simulink model "iLQCsimulation"  (R2025a)
settings: Solver=FixedStepAuto  StartTime=0.0  StopTime=20  FixedStep=0.01  RelTol=1e-3
StopFcn:
  | fprintf("Done\n");
values from neighbouring files (symbols this model uses):
  cmd = permute(cat(3, theta_ff', permute(theta_fb, [3, 1, 2])), [2, 3, 1])    [run_iLQR_simulation.m]
undefined symbols (not defined in the file or in its folder): ics, it, params, sim_, WpNav_hdg, WpNav_pos, WpNav_spd
libraries: matrix_library x1, sharedutil x1, sharedtransform x1, dspinverses x1
settings Model: Creator=Cindio  LastModifiedBy=cfeng
settings DataIOCC: SignalLogging=off  DSMLogging=off  ReturnWorkspaceOutputs=off
settings ModelReferenceCC: EnableRefExpFcnMdlSchedulingChecks=on
settings RTWCC: GPUComputeCapability=3.5  DLArmComputeVersion=19.05

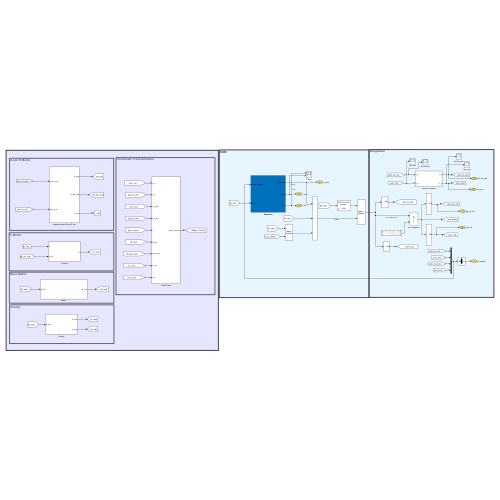
[thumbnail: Simulink's stored preview of the top-level diagram]
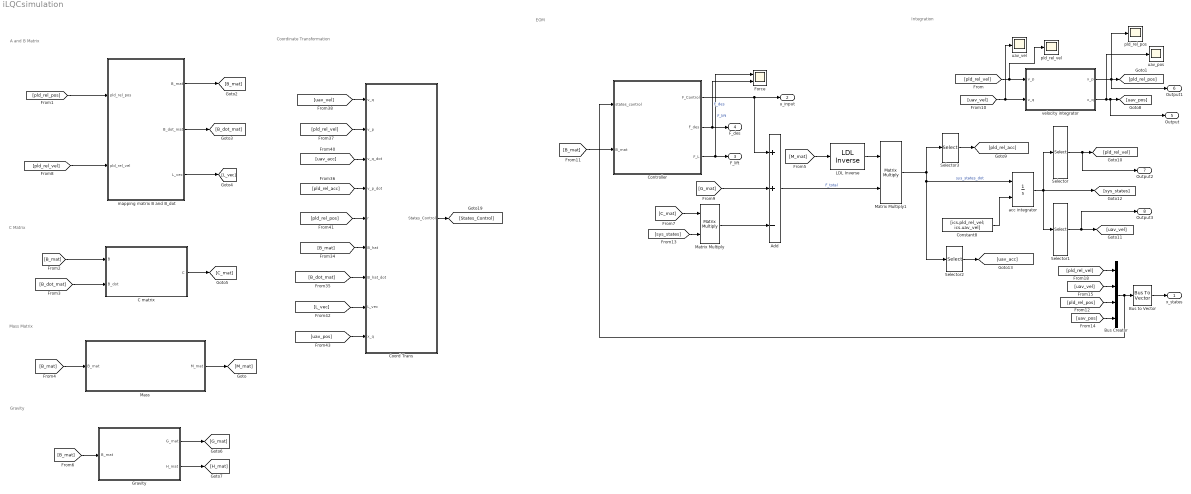
== system iLQCsimulation ==
  note: Integration
  note: EOM
  note: Gravity
  note: Mass Matrix
  note: C Matrix
  note: A and B Matrix
  note: Coordinate Transformation
  Add : Sum  Inputs=++-
  Bus Creator : BusCreator  Inputs=4
  Bus to Vector : BusToVector
  C matrix : Subsystem
  Constant8 : Constant  Value=[ics.pld_rel_vel; ics.uav_vel]  VectorParams1D=off
  Controller : Subsystem
  Coord Trans : Subsystem
  Force : Scope  NumInputPorts=2
      settings: ActiveDisplayYMinimum=-50.13137  ActiveDisplayYMaximum=10.24437
  Gravity : Subsystem
  LDL Inverse : dspinverses/LDL Inverse  errmode=Error
  Mass : Subsystem
  Matrix Multiply : Product  Multiplication=Matrix(*)
  Matrix Multiply1 : Product  Multiplication=Matrix(*)
  Selector : Selector  InputPortWidth=5  IndexOptions=Index vector (dialog)  Indices=[1 2]  OutputSizes=1
  Selector1 : Selector  InputPortWidth=5  IndexOptions=Index vector (dialog)  Indices=[3 4 5]  OutputSizes=1
  Selector2 : Selector  InputPortWidth=5  IndexOptions=Index vector (dialog)  Indices=[3 4 5]  OutputSizes=1
  Selector3 : Selector  InputPortWidth=5  IndexOptions=Index vector (dialog)  Indices=[1 2]  OutputSizes=1
  acc integrator : Integrator  InitialConditionSource=external
  mapping matrix B and B_dot : Subsystem
  pld_rel_pos : Scope
      settings: Title=Payload relative position  ActiveDisplayYMinimum=-0.0462  ActiveDisplayYMaximum=0.05217  YLabel=position (m)
  pld_rel_vel : Scope
      settings: Title=UAV Position  ActiveDisplayYMinimum=-0.10534  ActiveDisplayYMaximum=0.12291  YLabel=position (m)
  uav_pos : Scope
      settings: Title=UAV Position  ActiveDisplayYMinimum=-3.62298  ActiveDisplayYMaximum=2.12156  YLabel=position (m)  DataLoggingVariableName=ScopeData2
  uav_vel : Scope
      settings: Title=UAV Velocity  ActiveDisplayYMinimum=-0.42187  ActiveDisplayYMaximum=0.54304  YLabel=speed (m/s)  DataLoggingVariableName=ScopeData2
  velocity integrator : Subsystem
  x_states : Outport  SignalName=all_states
  u_input : Outport  Port=2  SignalName=u_input
  F_lift : Outport  Port=3  SignalName=F_lift
  F_des : Outport  Port=4  SignalName=F_des
  Output : Outport  Port=5  SignalName=uav_pos
  Output1 : Outport  Port=6  SignalName=pld_rel_pos
  Output2 : Outport  Port=7  SignalName=pld_rel_vel
  Output3 : Outport  Port=8  SignalName=uav_vel
  wires:
  [pld_rel_vel] -> pld_rel_vel/1, velocity integrator/1(v_p)
  velocity integrator/1(x_p) -> Output1/1, pld_rel_pos/1, [pld_rel_pos]
  mapping matrix B and B_dot/1(B_mat) -> [B_mat]
  mapping matrix B and B_dot/2(B_dot_mat) -> [B_dot_mat]
  mapping matrix B and B_dot/3(L_vec) -> [L_vec]
  [B_dot_mat] -> C matrix/2(B_dot)
  C matrix/1(C) -> [C_mat]
  [B_mat] -> Mass/1(B_mat)
  Mass/1(M_mat) -> [M_mat]
  [M_mat] -> LDL Inverse/1
  [B_mat] -> Gravity/1(B_mat)
  Gravity/2(H_mat) -> [H_mat]
  Matrix Multiply/1 -> Add/3
  [G_mat] -> Add/2
  Gravity/1(G_mat) -> [G_mat]
  [pld_rel_pos] -> mapping matrix B and B_dot/1(pld_rel_pos)
  [C_mat] -> Matrix Multiply/1
  [pld_rel_vel] -> mapping matrix B and B_dot/2(pld_rel_vel)
  [uav_vel] -> uav_vel/1, velocity integrator/2(v_q)
  [sys_states] -> Matrix Multiply/2
  LDL Inverse/1 -> Matrix Multiply1/1
  Add/1 -> Matrix Multiply1/2  "F_total"
  Matrix Multiply1/1 -> Selector3/1, Selector2/1, acc integrator/1  "sys_states_dot"
  Constant8/1 -> acc integrator/2
  acc integrator/1 -> Selector1/1, [sys_states], Selector/1
  Selector/1 -> Output2/1, [pld_rel_vel]
  Selector1/1 -> Output3/1, [uav_vel]
  [B_dot_mat] -> Coord Trans/7(B_hat_dot)
  [uav_vel] -> Coord Trans/1(v_q)
  [pld_rel_vel] -> Coord Trans/2(v_p)
  Coord Trans/1(States_Control) -> [States_Control]
  [B_mat] -> Coord Trans/6(B_hat)
  [pld_rel_pos] -> Coord Trans/5(r)
  [uav_pos] -> Coord Trans/9(x_q)
  [L_vec] -> Coord Trans/8(L_vec)
  [uav_acc] -> Coord Trans/3(v_q_dot)
  [pld_rel_acc] -> Coord Trans/4(v_p_dot)
  Selector3/1 -> [pld_rel_acc]
  Selector2/1 -> [uav_acc]
  Bus Creator/1 -> Bus to Vector/1, Controller/1(states_control)
  Controller/1(F_Control) -> Add/1, u_input/1
  velocity integrator/2(x_q) -> uav_pos/1, Output/1, [uav_pos]
  [pld_rel_pos] -> Bus Creator/3
  [uav_pos] -> Bus Creator/4
  [uav_vel] -> Bus Creator/2
  [pld_rel_vel] -> Bus Creator/1
  Bus to Vector/1 -> x_states/1
  [B_mat] -> Controller/2(B_mat)
  Controller/3(F_L) -> Force/1, F_lift/1  "F_lift"
  Controller/2(F_des) -> Force/2, F_des/1  "F_des"
  [B_mat] -> C matrix/1(B)

== system iLQCsimulation/C matrix ==
  B : Inport
  B_dot : Inport  Port=2
  Constant : Constant  Value=[zeros(2,3);zeros(3)]  VectorParams1D=off
  Matrix Concatenate : Concatenate  Mode=Multidimensional array  ConcatenateDimension=2
  Matrix Concatenate1 : Concatenate  Mode=Multidimensional array
  Matrix Multiply : Product  Multiplication=Matrix(*)
  Multiply : Gain  Gain=params.pld_mass
  Transpose : Math  Operator=transpose
  C : Outport
  wires:
  Constant/1 -> Matrix Concatenate/2
  Matrix Concatenate/1 -> C/1
  Matrix Multiply/1 -> Matrix Concatenate1/1
  B/1 -> Transpose/1
  Transpose/1 -> Matrix Multiply/1
  B_dot/1 -> Matrix Concatenate1/2, Matrix Multiply/2
  Multiply/1 -> Matrix Concatenate/1
  Matrix Concatenate1/1 -> Multiply/1

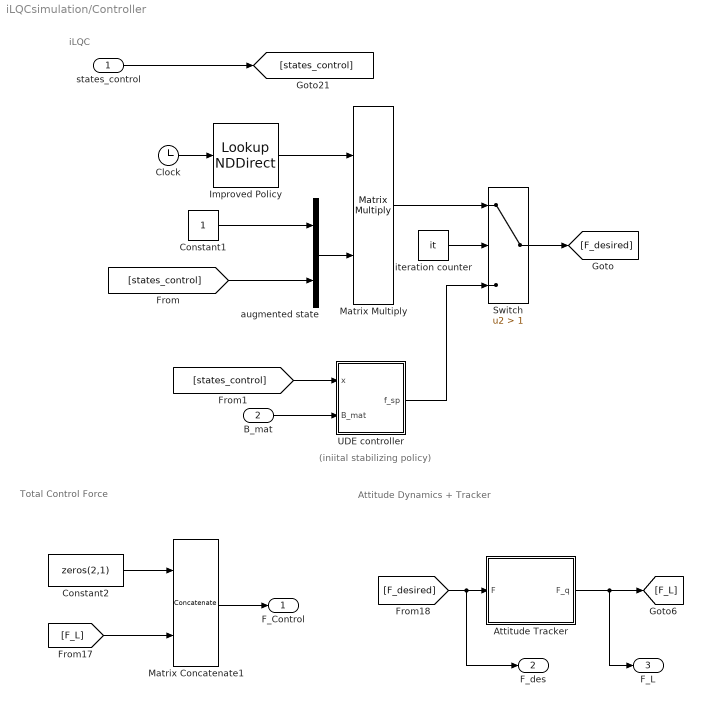
== system iLQCsimulation/Controller ==
  note: (iniital stabilizing policy)
  note: iLQC
  note: Total Control Force
  note: Attitude Dynamics + Tracker
  states_control : Inport
  B_mat : Inport  Port=2
  Attitude Tracker : Subsystem
  Clock : Clock
  Constant1 : Constant
  Constant2 : Constant  Value=zeros(2,1)
  Improved Policy : LookupNDDirect  NumberOfTableDimensions=3  InputsSelectThisObjectFromTable=2-D Matrix  Table=cmd  DiagnosticForOutOfRangeInput=Error
  Matrix Concatenate1 : Concatenate  Mode=Multidimensional array
  Matrix Multiply : Product  Multiplication=Matrix(*)
  Switch : Switch  Criteria=u2 > Threshold  Threshold=1  SaturateOnIntegerOverflow=off  InputSameDT=off
  "UDE controller " : Subsystem
  augmented state : Concatenate
  iteration counter : Constant  Value=it
  F_Control : Outport  VectorParamsAs1DForOutWhenUnconnected=off
  F_des : Outport  Port=2  VectorParamsAs1DForOutWhenUnconnected=off
  F_L : Outport  Port=3  VectorParamsAs1DForOutWhenUnconnected=off
  wires:
  Constant2/1 -> Matrix Concatenate1/1
  Matrix Concatenate1/1 -> F_Control/1
  [F_L] -> Matrix Concatenate1/2
  Attitude Tracker/1(F_q) -> F_L/1, [F_L]
  [F_desired] -> F_des/1, Attitude Tracker/1(F)
  Improved Policy/1 -> Matrix Multiply/1
  Clock/1 -> Improved Policy/1
  Matrix Multiply/1 -> Switch/1
  Constant1/1 -> augmented state/1
  iteration counter/1 -> Switch/2
  Switch/1 -> [F_desired]
  [states_control] -> "UDE controller "/1(x)
  B_mat/1 -> "UDE controller "/2(B_mat)
  "UDE controller "/1(f_sp) -> Switch/3
  states_control/1 -> [states_control]
  [states_control] -> augmented state/2
  augmented state/1 -> Matrix Multiply/2

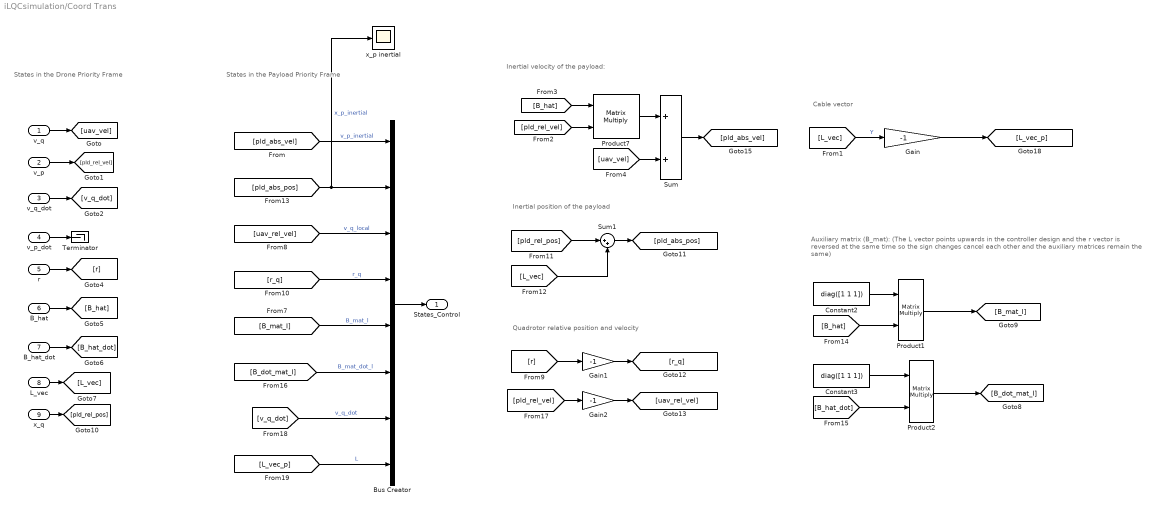
== system iLQCsimulation/Coord Trans ==
  note: Quadrotor relative position and velocity
  note: Auxiliary matrix (B_mat):
      | (The L vector points upwards in the controller design and the r vector is reversed at the same time so the sign changes cancel each other and the auxiliary matrices remain the same)
  note: Inertial position of the payload
  note: Cable vector
  note: Inertial velocity of the payload:
  note: States in the Drone Priority Frame
  note: States in the Payload Priority Frame
  v_q : Inport
  v_p : Inport  Port=2
  v_q_dot : Inport  Port=3
  v_p_dot : Inport  Port=4
  r : Inport  Port=5
  B_hat : Inport  Port=6
  B_hat_dot : Inport  Port=7
  L_vec : Inport  Port=8
  x_q : Inport  Port=9
  Bus Creator : BusCreator  Inputs=8
  Constant2 : Constant  Value=diag([1 1 1])
  Constant3 : Constant  Value=diag([1 1 1])
  Gain : Gain  Gain=-1
  Gain1 : Gain  Gain=-1
  Gain2 : Gain  Gain=-1
  Product1 : Product  Multiplication=Matrix(*)
  Product2 : Product  Multiplication=Matrix(*)
  Product7 : Product  Multiplication=Matrix(*)
  Sum : Sum
  Sum1 : Sum  Inputs=|++
  Terminator : Terminator
  x_p inertial : Scope
      settings: ActiveDisplayYMinimum=-3.375  ActiveDisplayYMaximum=0.375
  States_Control : Outport  VectorParamsAs1DForOutWhenUnconnected=off
  wires:
  Bus Creator/1 -> States_Control/1
  Product7/1 -> Sum/1
  Sum/1 -> [pld_abs_vel]
  [uav_vel] -> Sum/2
  [L_vec] -> Gain/1  "Y"
  Gain/1 -> [L_vec_p]
  v_q/1 -> [uav_vel]
  v_p/1 -> [pld_rel_vel]
  v_q_dot/1 -> [v_q_dot]
  v_p_dot/1 -> Terminator/1
  r/1 -> [r]
  B_hat/1 -> [B_hat]
  B_hat_dot/1 -> [B_hat_dot]
  L_vec/1 -> [L_vec]
  x_q/1 -> [pld_rel_pos]
  [pld_rel_pos] -> Sum1/1
  [L_vec] -> Sum1/2
  Sum1/1 -> [pld_abs_pos]
  [r] -> Gain1/1
  Gain1/1 -> [r_q]
  [pld_abs_vel] -> Bus Creator/1  "v_p_inertial"
  [pld_abs_pos] -> x_p inertial/1, Bus Creator/2  "x_p_inertial"
  [uav_rel_vel] -> Bus Creator/3  "v_q_local"
  [r_q] -> Bus Creator/4  "r_q"
  [B_mat_I] -> Bus Creator/5  "B_mat_l"
  [B_dot_mat_I] -> Bus Creator/6  "B_mat_dot_l"
  [B_hat] -> Product1/2
  Product1/1 -> [B_mat_I]
  [B_hat_dot] -> Product2/2
  Product2/1 -> [B_dot_mat_I]
  [pld_rel_vel] -> Gain2/1
  Gain2/1 -> [uav_rel_vel]
  [v_q_dot] -> Bus Creator/7  "v_q_dot"
  [L_vec_p] -> Bus Creator/8  "L"
  [pld_rel_vel] -> Product7/2
  [B_hat] -> Product7/1
  Constant2/1 -> Product1/1
  Constant3/1 -> Product2/1

== system iLQCsimulation/Gravity ==
  B_mat : Inport
  Constant : Constant  Value=zeros(2,3)  VectorParams1D=off
  Constant1 : Constant  Value=[eye(3),eye(3)]  VectorParams1D=off
  Constant2 : Constant  Value=params.derived.uav_weight
  Constant3 : Constant  Value=params.derived.pld_weight
  Matrix Concatenate : Concatenate  Mode=Multidimensional array  ConcatenateDimension=2
  Matrix Concatenate1 : Concatenate  Mode=Multidimensional array
  Matrix Concatenate2 : Concatenate
  Matrix Multiply : Product  Multiplication=Matrix(*)
  Transpose : Math  Operator=transpose
  G_mat : Outport
  H_mat : Outport  Port=2
  wires:
  Constant/1 -> Matrix Concatenate/2
  B_mat/1 -> Transpose/1
  Matrix Concatenate/1 -> Matrix Concatenate1/1
  Constant1/1 -> Matrix Concatenate1/2
  Matrix Concatenate1/1 -> [H], H_mat/1
  [H] -> Matrix Multiply/1
  Matrix Multiply/1 -> G_mat/1
  Matrix Concatenate2/1 -> Matrix Multiply/2
  Constant3/1 -> Matrix Concatenate2/1
  Transpose/1 -> Matrix Concatenate/1
  Constant2/1 -> Matrix Concatenate2/2

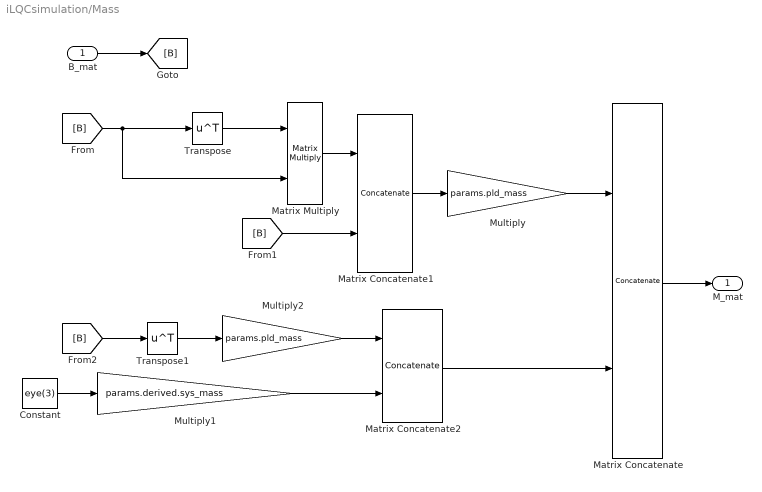
== system iLQCsimulation/Mass ==
  B_mat : Inport
  Constant : Constant  Value=eye(3)
  Matrix Concatenate : Concatenate  Mode=Multidimensional array  ConcatenateDimension=2
  Matrix Concatenate1 : Concatenate  Mode=Multidimensional array
  Matrix Concatenate2 : Concatenate  Mode=Multidimensional array
  Matrix Multiply : Product  Multiplication=Matrix(*)
  Multiply : Gain  Gain=params.pld_mass
  Multiply1 : Gain  Gain=params.derived.sys_mass
  Multiply2 : Gain  Gain=params.pld_mass
  Transpose : Math  Operator=transpose
  Transpose1 : Math  Operator=transpose
  M_mat : Outport
  wires:
  Matrix Concatenate/1 -> M_mat/1
  Matrix Concatenate1/1 -> Multiply/1
  Multiply/1 -> Matrix Concatenate/1
  B_mat/1 -> [B]
  [B] -> Matrix Multiply/2, Transpose/1
  Transpose/1 -> Matrix Multiply/1
  Matrix Multiply/1 -> Matrix Concatenate1/1
  [B] -> Matrix Concatenate1/2
  Constant/1 -> Multiply1/1
  Multiply1/1 -> Matrix Concatenate2/2
  Matrix Concatenate2/1 -> Matrix Concatenate/2
  [B] -> Transpose1/1
  Transpose1/1 -> Multiply2/1
  Multiply2/1 -> Matrix Concatenate2/1

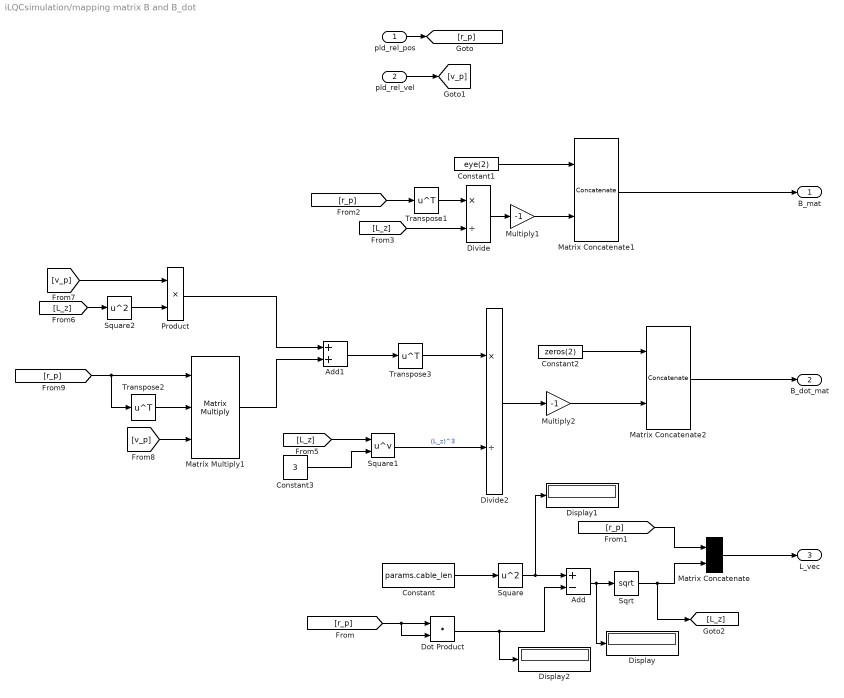
== system iLQCsimulation/mapping matrix B and B_dot ==
  pld_rel_pos : Inport
  pld_rel_vel : Inport  Port=2
  Add : Sum  Inputs=+-
  Add1 : Sum
  Constant : Constant  Value=params.cable_len
  Constant1 : Constant  Value=eye(2)
  Constant2 : Constant  Value=zeros(2)
  Constant3 : Constant  Value=3
  Display : Display
  Display1 : Display
  Display2 : Display
  Divide : Product  Inputs=*/
  Divide2 : Product  Inputs=*/
  Dot Product : DotProduct  OutDataTypeStr=Inherit: Inherit via internal rule
  Matrix Concatenate : Concatenate
  Matrix Concatenate1 : Concatenate  Mode=Multidimensional array
  Matrix Concatenate2 : Concatenate  Mode=Multidimensional array
  Matrix Multiply1 : Product  Inputs=3  Multiplication=Matrix(*)
  Multiply1 : Gain  Gain=-1
  Multiply2 : Gain  Gain=-1
  Product : Product
  Sqrt : Sqrt
  Square : Math  Operator=square
  Square1 : Math  Operator=pow
  Square2 : Math  Operator=square
  Transpose1 : Math  Operator=transpose
  Transpose2 : Math  Operator=transpose
  Transpose3 : Math  Operator=transpose
  B_mat : Outport
  B_dot_mat : Outport  Port=2
  L_vec : Outport  Port=3
  wires:
  Constant/1 -> Square/1
  Square/1 -> Display1/1, Add/1
  pld_rel_pos/1 -> [r_p]
  Add/1 -> Display/1, Sqrt/1
  Sqrt/1 -> [L_z], Matrix Concatenate/2
  [r_p] -> Matrix Concatenate/1
  pld_rel_vel/1 -> [v_p]
  Matrix Concatenate/1 -> L_vec/1
  [r_p] -> Transpose1/1
  Transpose1/1 -> Divide/1
  Constant1/1 -> Matrix Concatenate1/1
  Divide/1 -> Multiply1/1
  [L_z] -> Divide/2
  Multiply1/1 -> Matrix Concatenate1/2
  Matrix Concatenate1/1 -> B_mat/1
  Matrix Concatenate2/1 -> B_dot_mat/1
  Constant2/1 -> Matrix Concatenate2/1
  [L_z] -> Square1/1
  Square1/1 -> Divide2/2  "(L_z)^3"
  [L_z] -> Square2/1
  [v_p] -> Product/1
  Transpose2/1 -> Matrix Multiply1/2
  Matrix Multiply1/1 -> Add1/2
  [r_p] -> Transpose2/1, Matrix Multiply1/1
  [v_p] -> Matrix Multiply1/3
  Constant3/1 -> Square1/2
  Divide2/1 -> Multiply2/1
  Add1/1 -> Transpose3/1
  Product/1 -> Add1/1
  Square2/1 -> Product/2
  [r_p] -> Dot Product/2, Dot Product/1
  Dot Product/1 -> Display2/1, Add/2
  Transpose3/1 -> Divide2/1
  Multiply2/1 -> Matrix Concatenate2/2

== system iLQCsimulation/velocity integrator ==
  v_p : Inport
  v_q : Inport  Port=2
  Constant : Constant  Value=ics.pld_rel_pos
  Constant1 : Constant  Value=ics.uav_pos
  Integrator : Integrator  InitialConditionSource=external
  Integrator1 : Integrator  InitialConditionSource=external
  x_p : Outport
  x_q : Outport  Port=2
  wires:
  Integrator/1 -> x_p/1
  Constant/1 -> Integrator/2
  v_p/1 -> Integrator/1
  Constant1/1 -> Integrator1/2
  v_q/1 -> Integrator1/1
  Integrator1/1 -> x_q/1

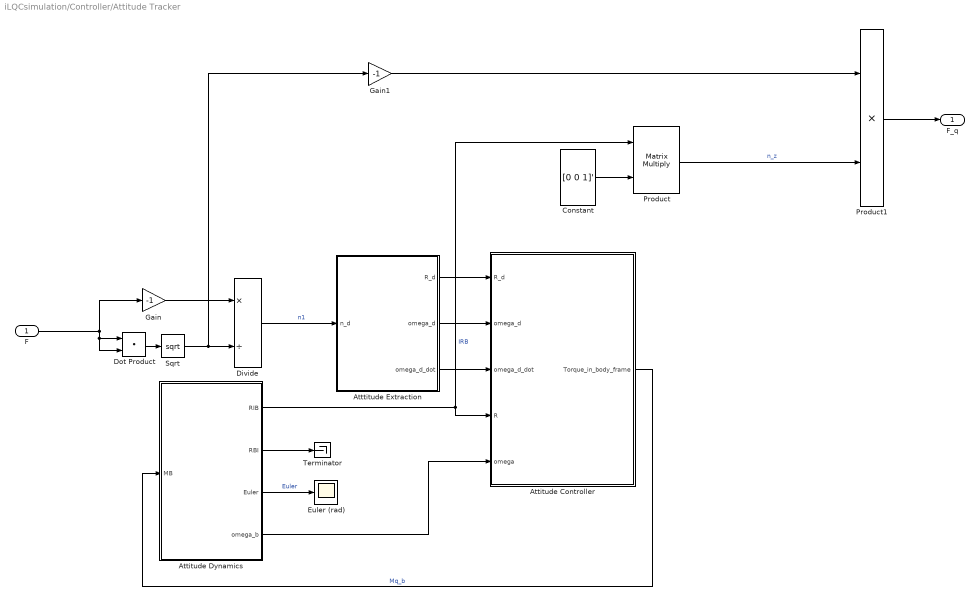
== system iLQCsimulation/Controller/Attitude Tracker ==
  F : Inport
  Attitude Controller : Subsystem
  Attitude Dynamics : Subsystem
  Atttitude Extraction : Subsystem
  Constant : Constant  Value=[0 0 1]'  VectorParams1D=off
  Divide : Product  Inputs=*/
  Dot Product : DotProduct  OutDataTypeStr=Inherit: Inherit via internal rule
  Euler (rad) : Scope
      settings: ActiveDisplayYMinimum=-0.01904  ActiveDisplayYMaximum=0.02201  DataLoggingVariableName=ScopeData2
  Gain : Gain  Gain=-1
  Gain1 : Gain  Gain=-1
  Product : Product  Multiplication=Matrix(*)
  Product1 : Product
  Sqrt : Sqrt
  Terminator : Terminator
  F_q : Outport  VectorParamsAs1DForOutWhenUnconnected=off
  wires:
  Constant/1 -> Product/2
  Product/1 -> Product1/2  "n_z"
  Product1/1 -> F_q/1
  Dot Product/1 -> Sqrt/1
  Atttitude Extraction/1(R_d) -> Attitude Controller/1(R_d)
  Atttitude Extraction/2(omega_d) -> Attitude Controller/2(omega_d)
  Atttitude Extraction/3(omega_d_dot) -> Attitude Controller/3(omega_d_dot)
  Divide/1 -> Atttitude Extraction/1(n_d)  "n1"
  Attitude Dynamics/4(omega_b) -> Attitude Controller/5(omega)
  Attitude Dynamics/3(Euler) -> Euler (rad)/1  "Euler"
  Attitude Dynamics/2(RBI) -> Terminator/1
  Attitude Dynamics/1(RIB) -> Attitude Controller/4(R), Product/1  "IRB"
  Attitude Controller/1(Torque_in_body_frame) -> Attitude Dynamics/1(MB)  "Mq_b"
  F/1 -> Gain/1, Dot Product/2, Dot Product/1
  Sqrt/1 -> Gain1/1, Divide/2
  Gain/1 -> Divide/1
  Gain1/1 -> Product1/1

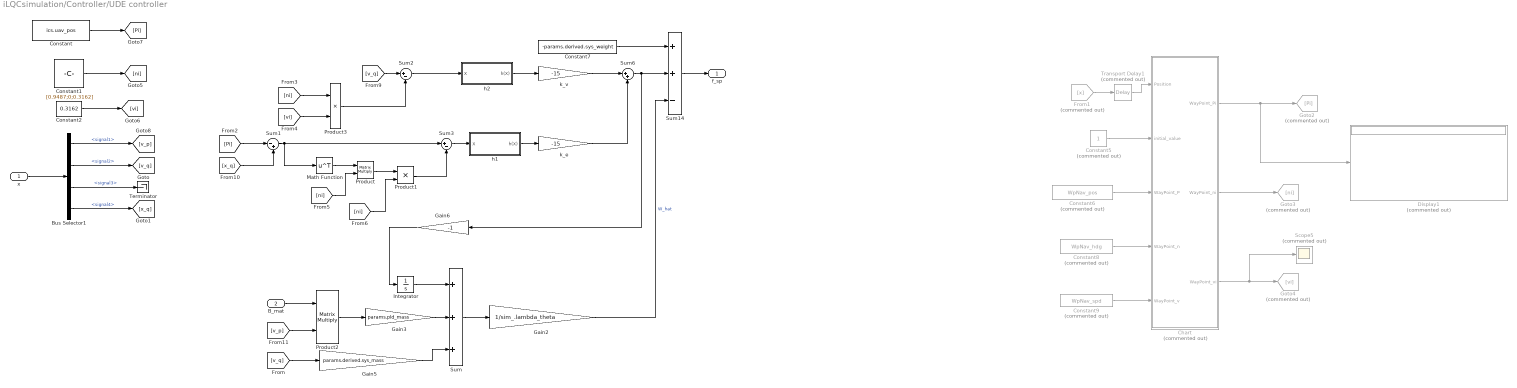
== system iLQCsimulation/Controller/UDE controller  ==
  x : Inport
  B_mat : Inport  Port=2
  Bus Selector1 : BusSelector  OutputSignals=signal1,signal2,signal3,signal4
  Chart : Stateflow chart  Commented=on  TreatAsAtomicUnit=on
  Constant : Constant  Value=ics.uav_pos  VectorParams1D=off
  Constant1 : Constant  Value=[0.9487;0;0.3162]  VectorParams1D=off
  Constant2 : Constant  Value=0.3162
  Constant5 : Constant  Commented=on
  Constant6 : Constant  Commented=on  Value=WpNav_pos
  Constant7 : Constant  Value=-params.derived.sys_weight  VectorParams1D=off
  Constant8 : Constant  Commented=on  Value=WpNav_hdg
  Constant9 : Constant  Commented=on  Value=WpNav_spd
  Display1 : Display  Commented=on
  From1 : From  Commented=on  GotoTag=x
  Gain2 : Gain  Gain=1/sim_.lambda_theta
  Gain3 : Gain  Gain=params.pld_mass
  Gain5 : Gain  Gain=params.derived.sys_mass
  Gain6 : Gain  Gain=-1
  Goto2 : Goto  Commented=on  GotoTag=Pi
  Goto3 : Goto  Commented=on  GotoTag=ni
  Goto4 : Goto  Commented=on  GotoTag=vi
  Integrator : Integrator
  Math Function : Math  Operator=transpose  SignedPower=on
  Product : Product  Multiplication=Matrix(*)
  Product1 : Product
  Product2 : Product  Multiplication=Matrix(*)
  Product3 : Product
  Scope5 : Scope  Commented=on
      settings: ActiveDisplayYMinimum=-1.25  ActiveDisplayYMaximum=11.25  DataLoggingVariableName=ScopeData3
  Sum : Sum  Inputs=+++
  Sum1 : Sum  Inputs=|-+
  Sum14 : Sum  Inputs=++-
  Sum2 : Sum  Inputs=|+-
  Sum3 : Sum  Inputs=|+-
  Sum6 : Sum  Inputs=|++
  Terminator : Terminator
  Transport Delay1 : TransportDelay  Commented=on  DelayTime=0.3
  h1 : Subsystem
  h2 : Subsystem
  k_e : Gain  Gain=-15
  k_v : Gain  Gain=-15
  f_sp : Outport
  wires:
  Sum14/1 -> f_sp/1
  [ni] -> Product3/1
  [Pi] -> Sum1/1
  Product3/1 -> Sum2/2
  h1/1(h(X)) -> k_e/1
  k_e/1 -> Sum6/2
  Sum1/1 -> Math Function/1, Sum3/1
  Math Function/1 -> Product/1
  [ni] -> Product/2
  Product/1 -> Product1/1
  [ni] -> Product1/2
  Product1/1 -> Sum3/2
  k_v/1 -> Sum6/1
  h2/1(h(X)) -> k_v/1
  Sum2/1 -> h2/1(X)
  Sum6/1 -> Gain6/1, Sum14/2
  Constant7/1 -> Sum14/1
  Sum/1 -> Gain2/1
  Bus Selector1/1 -> [v_p]  "<signal1>"
  Product2/1 -> Gain3/1
  [v_q] -> Gain5/1
  Gain3/1 -> Sum/2
  Gain5/1 -> Sum/3
  Integrator/1 -> Sum/1
  Gain6/1 -> Integrator/1
  Gain2/1 -> Sum14/3  "W_hat"
  Constant5/1 -> Chart/2(initial_value)
  From1/1 -> Transport Delay1/1
  Constant6/1 -> Chart/3(WayPoint_P)
  Constant8/1 -> Chart/4(WayPoint_n)
  Constant9/1 -> Chart/5(WayPoint_v)
  [vi] -> Product3/2
  Transport Delay1/1 -> Chart/1(Position)
  Sum3/1 -> h1/1(X)
  Chart/2(WayPoint_ni) -> Goto3/1
  Chart/3(WayPoint_vi) -> Scope5/1, Goto4/1
  Chart/1(WayPoint_Pi) -> Display1/1, Goto2/1
  Bus Selector1/3 -> Terminator/1  "<signal3>"
  x/1 -> Bus Selector1/1
  Constant/1 -> [Pi]
  Constant1/1 -> [ni]
  Constant2/1 -> [vi]
  B_mat/1 -> Product2/1
  Bus Selector1/2 -> [v_q]  "<signal2>"
  [v_q] -> Sum2/1
  Bus Selector1/4 -> [x_q]  "<signal4>"
  [x_q] -> Sum1/2
  [v_p] -> Product2/2

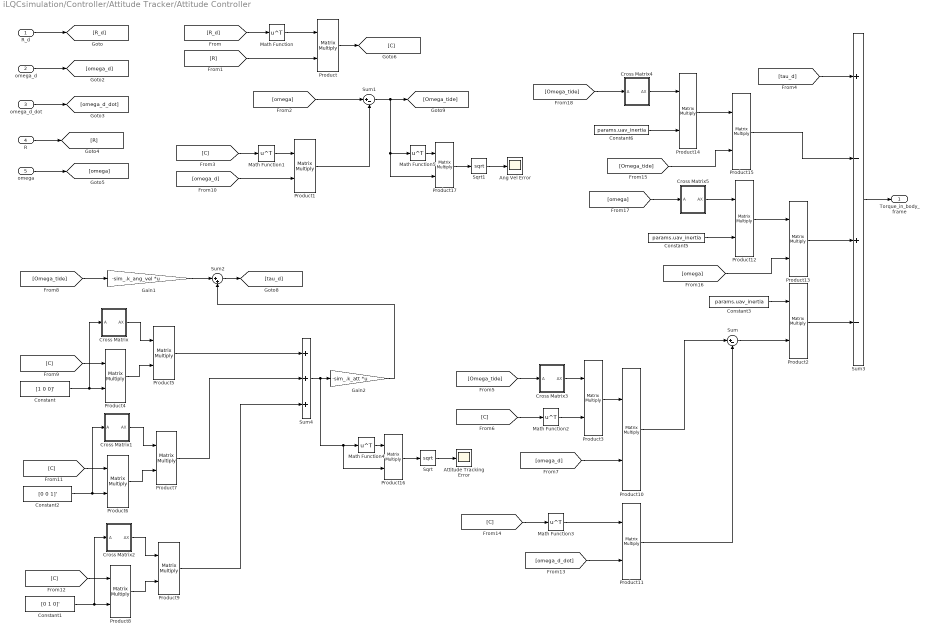
== system iLQCsimulation/Controller/Attitude Tracker/Attitude Controller ==
  R_d : Inport
  omega_d : Inport  Port=2
  omega_d_dot : Inport  Port=3
  R : Inport  Port=4
  omega : Inport  Port=5
  Ang Vel Error : Scope
      settings: ActiveDisplayYMinimum=-1.77018  ActiveDisplayYMaximum=15.93169  DataLoggingVariableName=ScopeData9
  Attitude Tracking Error : Scope
      settings: ActiveDisplayYMinimum=-0.14827  ActiveDisplayYMaximum=1.33442  DataLoggingVariableName=ScopeData10
  Constant : Constant  Value=[1 0 0]'
  Constant1 : Constant  Value=[0 1 0]'
  Constant2 : Constant  Value=[0 0 1]'
  Constant3 : Constant  Value=params.uav_inertia  VectorParams1D=off
  Constant5 : Constant  Value=params.uav_inertia  VectorParams1D=off
  Constant6 : Constant  Value=params.uav_inertia  VectorParams1D=off
  Cross Matrix : Subsystem
  Cross Matrix1 : Subsystem
  Cross Matrix2 : Subsystem
  Cross Matrix3 : Subsystem
  Cross Matrix4 : Subsystem
  Cross Matrix5 : Subsystem
  Gain1 : Gain  Gain=-sim_.k_ang_vel  Multiplication=Matrix(K*u)
  Gain2 : Gain  Gain=-sim_.k_att  Multiplication=Matrix(K*u)
  Math Function{,1..5} (6 alike) : Math  Operator=transpose  SignedPower=on
  Product{,1..17} (18 alike) : Product  Multiplication=Matrix(*)
  Sqrt : Sqrt
  Sqrt1 : Sqrt
  Sum : Sum  Inputs=|+-
  Sum1 : Sum  Inputs=|+-
  Sum2 : Sum  Inputs=|++
  Sum3 : Sum  Inputs=+-+-
  Sum4 : Sum  Inputs=+++
  Torque_in_body_frame : Outport  VectorParamsAs1DForOutWhenUnconnected=off
  wires:
  R_d/1 -> [R_d]
  omega_d/1 -> [omega_d]
  omega_d_dot/1 -> [omega_d_dot]
  [R_d] -> Math Function/1
  Math Function/1 -> Product/1
  R/1 -> [R]
  omega/1 -> [omega]
  [R] -> Product/2
  Product/1 -> [C]
  [C] -> Math Function1/1
  Math Function1/1 -> Product1/1
  [omega] -> Sum1/1
  Product1/1 -> Sum1/2
  [omega_d] -> Product1/2
  Sum2/1 -> [tau_d]
  Gain1/1 -> Sum2/1
  [Omega_tide] -> Gain1/1
  [tau_d] -> Sum3/1
  [C] -> Product4/1
  Constant/1 -> Cross Matrix/1(A), Product4/2
  Cross Matrix/1(AX) -> Product5/1
  Product4/1 -> Product5/2
  [C] -> Product6/1
  Constant2/1 -> Cross Matrix1/1(A), Product6/2
  Cross Matrix1/1(AX) -> Product7/1
  Product6/1 -> Product7/2
  Product7/1 -> Sum4/2
  [C] -> Product8/1
  Constant1/1 -> Cross Matrix2/1(A), Product8/2
  Cross Matrix2/1(AX) -> Product9/1
  Product8/1 -> Product9/2
  Product9/1 -> Sum4/3
  Product5/1 -> Sum4/1
  Gain2/1 -> Sum2/2
  Sum3/1 -> Torque_in_body_frame/1
  Constant3/1 -> Product2/1
  Sum/1 -> Product2/2
  [Omega_tide] -> Cross Matrix3/1(A)
  [C] -> Math Function2/1
  Cross Matrix3/1(AX) -> Product3/1
  Math Function2/1 -> Product3/2
  Product3/1 -> Product10/1
  [omega_d] -> Product10/2
  Product10/1 -> Sum/1
  [C] -> Math Function3/1
  Math Function3/1 -> Product11/1
  [omega_d_dot] -> Product11/2
  Product11/1 -> Sum/2
  Product2/1 -> Sum3/4
  Product13/1 -> Sum3/3
  Product12/1 -> Product13/1
  [omega] -> Product13/2
  [omega] -> Cross Matrix5/1(A)
  Cross Matrix5/1(AX) -> Product12/1
  Constant5/1 -> Product12/2
  Product14/1 -> Product15/1
  [Omega_tide] -> Product15/2
  [Omega_tide] -> Cross Matrix4/1(A)
  Cross Matrix4/1(AX) -> Product14/1
  Constant6/1 -> Product14/2
  Product15/1 -> Sum3/2
  Sum4/1 -> Product16/2, Math Function4/1, Gain2/1
  Math Function4/1 -> Product16/1
  Product16/1 -> Sqrt/1
  Sqrt/1 -> Attitude Tracking Error/1
  Sum1/1 -> Math Function5/1, Product17/2, [Omega_tide]
  Math Function5/1 -> Product17/1
  Product17/1 -> Sqrt1/1
  Sqrt1/1 -> Ang Vel Error/1

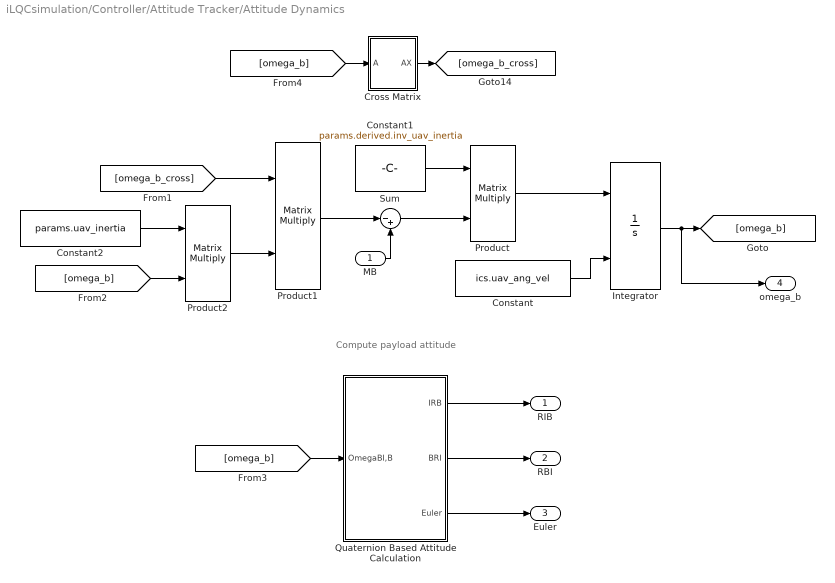
== system iLQCsimulation/Controller/Attitude Tracker/Attitude Dynamics ==
  note: Compute payload attitude
  MB : Inport
  Constant : Constant  Value=ics.uav_ang_vel  VectorParams1D=off
  Constant1 : Constant  Value=params.derived.inv_uav_inertia  VectorParams1D=off
  Constant2 : Constant  Value=params.uav_inertia  VectorParams1D=off
  Cross Matrix : Subsystem
  Integrator : Integrator  InitialConditionSource=external
  Product : Product  Multiplication=Matrix(*)
  Product1 : Product  Multiplication=Matrix(*)
  Product2 : Product  Multiplication=Matrix(*)
  Quaternion Based Attitude Calculation : Subsystem
  Sum : Sum  Inputs=|-+
  RIB : Outport  VectorParamsAs1DForOutWhenUnconnected=off
  RBI : Outport  Port=2  VectorParamsAs1DForOutWhenUnconnected=off
  Euler : Outport  Port=3  VectorParamsAs1DForOutWhenUnconnected=off
  omega_b : Outport  Port=4  VectorParamsAs1DForOutWhenUnconnected=off
  wires:
  [omega_b] -> Cross Matrix/1(A)
  Cross Matrix/1(AX) -> [omega_b_cross]
  [omega_b] -> Quaternion Based Attitude Calculation/1(OmegaBI,B)
  Quaternion Based Attitude Calculation/1(IRB) -> RIB/1
  Quaternion Based Attitude Calculation/2(BRI) -> RBI/1
  Quaternion Based Attitude Calculation/3(Euler) -> Euler/1
  Integrator/1 -> omega_b/1, [omega_b]
  Constant/1 -> Integrator/2
  Product/1 -> Integrator/1
  Constant1/1 -> Product/1
  Sum/1 -> Product/2
  MB/1 -> Sum/2
  [omega_b_cross] -> Product1/1
  Product2/1 -> Product1/2
  Constant2/1 -> Product2/1
  [omega_b] -> Product2/2
  Product1/1 -> Sum/1

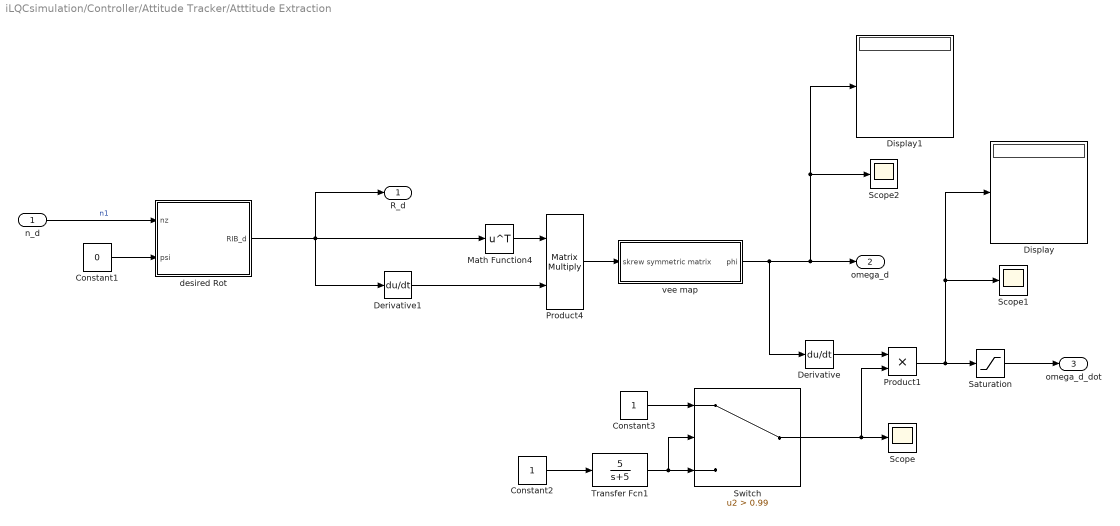
== system iLQCsimulation/Controller/Attitude Tracker/Atttitude Extraction ==
  n_d : Inport
  Constant1 : Constant  Value=0
  Constant2 : Constant
  Constant3 : Constant
  Derivative : Derivative
  Derivative1 : Derivative
  Display : Display
  Display1 : Display
  Math Function4 : Math  Operator=transpose  SignedPower=on
  Product1 : Product
  Product4 : Product  Multiplication=Matrix(*)
  Saturation : Saturate  UpperLimit=10  LowerLimit=-10
  Scope : Scope
      settings: ActiveDisplayYMinimum=0.99987  ActiveDisplayYMaximum=1.00016  DataLoggingVariableName=ScopeData3
  Scope1 : Scope
      settings: ActiveDisplayYMinimum=-989.1974  ActiveDisplayYMaximum=1431.98918
  Scope2 : Scope
      settings: ActiveDisplayYMinimum=-1.34126  ActiveDisplayYMaximum=1.3459  DataLoggingVariableName=ScopeData2
  Switch : Switch  Criteria=u2 > Threshold  Threshold=0.99  ZeroCross=off  SaturateOnIntegerOverflow=off  InputSameDT=off
  Transfer Fcn1 : TransferFcn  Numerator=[5]  Denominator=[1 5]
  desired Rot : Subsystem
  vee map : Subsystem
  R_d : Outport  VectorParamsAs1DForOutWhenUnconnected=off
  omega_d : Outport  Port=2  VectorParamsAs1DForOutWhenUnconnected=off
  omega_d_dot : Outport  Port=3  VectorParamsAs1DForOutWhenUnconnected=off
  wires:
  Math Function4/1 -> Product4/1
  Derivative1/1 -> Product4/2
  Product4/1 -> vee map/1(skrew symmetric matrix)
  vee map/1(phi) -> Derivative/1, Display1/1, Scope2/1, omega_d/1
  n_d/1 -> desired Rot/1(nz)  "n1"
  Constant1/1 -> desired Rot/2(psi)
  desired Rot/1(RIB_d) -> Derivative1/1, Math Function4/1, R_d/1
  Constant2/1 -> Transfer Fcn1/1
  Derivative/1 -> Product1/1
  Product1/1 -> Display/1, Scope1/1, Saturation/1
  Switch/1 -> Scope/1, Product1/2
  Constant3/1 -> Switch/1
  Transfer Fcn1/1 -> Switch/2, Switch/3
  Saturation/1 -> omega_d_dot/1

== system iLQCsimulation/Controller/UDE controller /h1 ==
  X : Inport
  Divide : Product  Inputs=*/
  Math Function : Math  Operator=transpose  SignedPower=on
  Product : Product  Multiplication=Matrix(*)
  Sum : Sum  Inputs=|++
  c_x : Constant
  h(X) : Outport
  wires:
  X/1 -> Divide/1, Product/2, Math Function/1
  Math Function/1 -> Product/1
  Product/1 -> Sum/1
  c_x/1 -> Sum/2
  Sum/1 -> Divide/2
  Divide/1 -> h(X)/1

== system iLQCsimulation/Controller/UDE controller /h2 ==
  X : Inport
  Divide : Product  Inputs=*/
  Math Function : Math  Operator=transpose  SignedPower=on
  Product : Product  Multiplication=Matrix(*)
  Sum : Sum  Inputs=|++
  c_v : Constant
  h(X) : Outport
  wires:
  X/1 -> Divide/1, Product/2, Math Function/1
  Math Function/1 -> Product/1
  Product/1 -> Sum/1
  c_v/1 -> Sum/2
  Sum/1 -> Divide/2
  Divide/1 -> h(X)/1

== system iLQCsimulation/Controller/Attitude Tracker/Attitude Controller/Cross Matrix ==
  A : Inport
  Constant1 : Constant  Value=0  VectorParams1D=off
  Constant2 : Constant  Value=0  VectorParams1D=off
  Constant3 : Constant  Value=0  VectorParams1D=off
  Demux2 : Demux  Outputs=3
  Gain : Gain  Gain=-1
  Gain1 : Gain  Gain=-1
  Gain2 : Gain  Gain=-1
  Matrix Concatenate : Concatenate  NumInputs=3  Mode=Multidimensional array  ConcatenateDimension=2
  Matrix Concatenate1 : Concatenate  NumInputs=3  Mode=Multidimensional array
  Matrix Concatenate2 : Concatenate  NumInputs=3  Mode=Multidimensional array
  Matrix Concatenate3 : Concatenate  NumInputs=3  Mode=Multidimensional array
  AX : Outport  VectorParamsAs1DForOutWhenUnconnected=off
  wires:
  A/1 -> Demux2/1
  Demux2/1 -> Gain1/1, Matrix Concatenate2/3  "r1"
  Demux2/2 -> Gain2/1, Matrix Concatenate3/1  "r2"
  Matrix Concatenate/1 -> AX/1
  Demux2/3 -> Gain/1, Matrix Concatenate1/2  "r3"
  Matrix Concatenate1/1 -> Matrix Concatenate/1
  Matrix Concatenate2/1 -> Matrix Concatenate/2
  Constant2/1 -> Matrix Concatenate2/2
  Gain/1 -> Matrix Concatenate2/1
  Matrix Concatenate3/1 -> Matrix Concatenate/3
  Gain1/1 -> Matrix Concatenate3/2
  Constant3/1 -> Matrix Concatenate3/3
  Constant1/1 -> Matrix Concatenate1/1
  Gain2/1 -> Matrix Concatenate1/3

== system iLQCsimulation/Controller/Attitude Tracker/Attitude Controller/Cross Matrix1 ==
  A : Inport
  Constant1 : Constant  Value=0  VectorParams1D=off
  Constant2 : Constant  Value=0  VectorParams1D=off
  Constant3 : Constant  Value=0  VectorParams1D=off
  Demux2 : Demux  Outputs=3
  Gain : Gain  Gain=-1
  Gain1 : Gain  Gain=-1
  Gain2 : Gain  Gain=-1
  Matrix Concatenate : Concatenate  NumInputs=3  Mode=Multidimensional array  ConcatenateDimension=2
  Matrix Concatenate1 : Concatenate  NumInputs=3  Mode=Multidimensional array
  Matrix Concatenate2 : Concatenate  NumInputs=3  Mode=Multidimensional array
  Matrix Concatenate3 : Concatenate  NumInputs=3  Mode=Multidimensional array
  AX : Outport  VectorParamsAs1DForOutWhenUnconnected=off
  wires:
  A/1 -> Demux2/1
  Demux2/1 -> Gain1/1, Matrix Concatenate2/3  "r1"
  Demux2/2 -> Gain2/1, Matrix Concatenate3/1  "r2"
  Matrix Concatenate/1 -> AX/1
  Demux2/3 -> Gain/1, Matrix Concatenate1/2  "r3"
  Matrix Concatenate1/1 -> Matrix Concatenate/1
  Matrix Concatenate2/1 -> Matrix Concatenate/2
  Constant2/1 -> Matrix Concatenate2/2
  Gain/1 -> Matrix Concatenate2/1
  Matrix Concatenate3/1 -> Matrix Concatenate/3
  Gain1/1 -> Matrix Concatenate3/2
  Constant3/1 -> Matrix Concatenate3/3
  Constant1/1 -> Matrix Concatenate1/1
  Gain2/1 -> Matrix Concatenate1/3

== system iLQCsimulation/Controller/Attitude Tracker/Attitude Controller/Cross Matrix2 ==
  A : Inport
  Constant1 : Constant  Value=0  VectorParams1D=off
  Constant2 : Constant  Value=0  VectorParams1D=off
  Constant3 : Constant  Value=0  VectorParams1D=off
  Demux2 : Demux  Outputs=3
  Gain : Gain  Gain=-1
  Gain1 : Gain  Gain=-1
  Gain2 : Gain  Gain=-1
  Matrix Concatenate : Concatenate  NumInputs=3  Mode=Multidimensional array  ConcatenateDimension=2
  Matrix Concatenate1 : Concatenate  NumInputs=3  Mode=Multidimensional array
  Matrix Concatenate2 : Concatenate  NumInputs=3  Mode=Multidimensional array
  Matrix Concatenate3 : Concatenate  NumInputs=3  Mode=Multidimensional array
  AX : Outport  VectorParamsAs1DForOutWhenUnconnected=off
  wires:
  A/1 -> Demux2/1
  Demux2/1 -> Gain1/1, Matrix Concatenate2/3  "r1"
  Demux2/2 -> Gain2/1, Matrix Concatenate3/1  "r2"
  Matrix Concatenate/1 -> AX/1
  Demux2/3 -> Gain/1, Matrix Concatenate1/2  "r3"
  Matrix Concatenate1/1 -> Matrix Concatenate/1
  Matrix Concatenate2/1 -> Matrix Concatenate/2
  Constant2/1 -> Matrix Concatenate2/2
  Gain/1 -> Matrix Concatenate2/1
  Matrix Concatenate3/1 -> Matrix Concatenate/3
  Gain1/1 -> Matrix Concatenate3/2
  Constant3/1 -> Matrix Concatenate3/3
  Constant1/1 -> Matrix Concatenate1/1
  Gain2/1 -> Matrix Concatenate1/3

== system iLQCsimulation/Controller/Attitude Tracker/Attitude Controller/Cross Matrix3 ==
  A : Inport
  Constant1 : Constant  Value=0  VectorParams1D=off
  Constant2 : Constant  Value=0  VectorParams1D=off
  Constant3 : Constant  Value=0  VectorParams1D=off
  Demux2 : Demux  Outputs=3
  Gain : Gain  Gain=-1
  Gain1 : Gain  Gain=-1
  Gain2 : Gain  Gain=-1
  Matrix Concatenate : Concatenate  NumInputs=3  Mode=Multidimensional array  ConcatenateDimension=2
  Matrix Concatenate1 : Concatenate  NumInputs=3  Mode=Multidimensional array
  Matrix Concatenate2 : Concatenate  NumInputs=3  Mode=Multidimensional array
  Matrix Concatenate3 : Concatenate  NumInputs=3  Mode=Multidimensional array
  AX : Outport  VectorParamsAs1DForOutWhenUnconnected=off
  wires:
  A/1 -> Demux2/1
  Demux2/1 -> Gain1/1, Matrix Concatenate2/3  "r1"
  Demux2/2 -> Gain2/1, Matrix Concatenate3/1  "r2"
  Matrix Concatenate/1 -> AX/1
  Demux2/3 -> Gain/1, Matrix Concatenate1/2  "r3"
  Matrix Concatenate1/1 -> Matrix Concatenate/1
  Matrix Concatenate2/1 -> Matrix Concatenate/2
  Constant2/1 -> Matrix Concatenate2/2
  Gain/1 -> Matrix Concatenate2/1
  Matrix Concatenate3/1 -> Matrix Concatenate/3
  Gain1/1 -> Matrix Concatenate3/2
  Constant3/1 -> Matrix Concatenate3/3
  Constant1/1 -> Matrix Concatenate1/1
  Gain2/1 -> Matrix Concatenate1/3

== system iLQCsimulation/Controller/Attitude Tracker/Attitude Controller/Cross Matrix4 ==
  A : Inport
  Constant1 : Constant  Value=0  VectorParams1D=off
  Constant2 : Constant  Value=0  VectorParams1D=off
  Constant3 : Constant  Value=0  VectorParams1D=off
  Demux2 : Demux  Outputs=3
  Gain : Gain  Gain=-1
  Gain1 : Gain  Gain=-1
  Gain2 : Gain  Gain=-1
  Matrix Concatenate : Concatenate  NumInputs=3  Mode=Multidimensional array  ConcatenateDimension=2
  Matrix Concatenate1 : Concatenate  NumInputs=3  Mode=Multidimensional array
  Matrix Concatenate2 : Concatenate  NumInputs=3  Mode=Multidimensional array
  Matrix Concatenate3 : Concatenate  NumInputs=3  Mode=Multidimensional array
  AX : Outport  VectorParamsAs1DForOutWhenUnconnected=off
  wires:
  A/1 -> Demux2/1
  Demux2/1 -> Gain1/1, Matrix Concatenate2/3  "r1"
  Demux2/2 -> Gain2/1, Matrix Concatenate3/1  "r2"
  Matrix Concatenate/1 -> AX/1
  Demux2/3 -> Gain/1, Matrix Concatenate1/2  "r3"
  Matrix Concatenate1/1 -> Matrix Concatenate/1
  Matrix Concatenate2/1 -> Matrix Concatenate/2
  Constant2/1 -> Matrix Concatenate2/2
  Gain/1 -> Matrix Concatenate2/1
  Matrix Concatenate3/1 -> Matrix Concatenate/3
  Gain1/1 -> Matrix Concatenate3/2
  Constant3/1 -> Matrix Concatenate3/3
  Constant1/1 -> Matrix Concatenate1/1
  Gain2/1 -> Matrix Concatenate1/3

== system iLQCsimulation/Controller/Attitude Tracker/Attitude Controller/Cross Matrix5 ==
  A : Inport
  Constant1 : Constant  Value=0  VectorParams1D=off
  Constant2 : Constant  Value=0  VectorParams1D=off
  Constant3 : Constant  Value=0  VectorParams1D=off
  Demux2 : Demux  Outputs=3
  Gain : Gain  Gain=-1
  Gain1 : Gain  Gain=-1
  Gain2 : Gain  Gain=-1
  Matrix Concatenate : Concatenate  NumInputs=3  Mode=Multidimensional array  ConcatenateDimension=2
  Matrix Concatenate1 : Concatenate  NumInputs=3  Mode=Multidimensional array
  Matrix Concatenate2 : Concatenate  NumInputs=3  Mode=Multidimensional array
  Matrix Concatenate3 : Concatenate  NumInputs=3  Mode=Multidimensional array
  AX : Outport  VectorParamsAs1DForOutWhenUnconnected=off
  wires:
  A/1 -> Demux2/1
  Demux2/1 -> Gain1/1, Matrix Concatenate2/3  "r1"
  Demux2/2 -> Gain2/1, Matrix Concatenate3/1  "r2"
  Matrix Concatenate/1 -> AX/1
  Demux2/3 -> Gain/1, Matrix Concatenate1/2  "r3"
  Matrix Concatenate1/1 -> Matrix Concatenate/1
  Matrix Concatenate2/1 -> Matrix Concatenate/2
  Constant2/1 -> Matrix Concatenate2/2
  Gain/1 -> Matrix Concatenate2/1
  Matrix Concatenate3/1 -> Matrix Concatenate/3
  Gain1/1 -> Matrix Concatenate3/2
  Constant3/1 -> Matrix Concatenate3/3
  Constant1/1 -> Matrix Concatenate1/1
  Gain2/1 -> Matrix Concatenate1/3

== system iLQCsimulation/Controller/Attitude Tracker/Attitude Dynamics/Cross Matrix ==
  A : Inport
  Constant1 : Constant  Value=0  VectorParams1D=off
  Constant2 : Constant  Value=0  VectorParams1D=off
  Constant3 : Constant  Value=0  VectorParams1D=off
  Demux2 : Demux  Outputs=3
  Gain : Gain  Gain=-1
  Gain1 : Gain  Gain=-1
  Gain2 : Gain  Gain=-1
  Matrix Concatenate : Concatenate  NumInputs=3  Mode=Multidimensional array  ConcatenateDimension=2
  Matrix Concatenate1 : Concatenate  NumInputs=3  Mode=Multidimensional array
  Matrix Concatenate2 : Concatenate  NumInputs=3  Mode=Multidimensional array
  Matrix Concatenate3 : Concatenate  NumInputs=3  Mode=Multidimensional array
  AX : Outport  VectorParamsAs1DForOutWhenUnconnected=off
  wires:
  A/1 -> Demux2/1
  Demux2/1 -> Gain1/1, Matrix Concatenate2/3  "r1"
  Demux2/2 -> Gain2/1, Matrix Concatenate3/1  "r2"
  Matrix Concatenate/1 -> AX/1
  Demux2/3 -> Gain/1, Matrix Concatenate1/2  "r3"
  Matrix Concatenate1/1 -> Matrix Concatenate/1
  Matrix Concatenate2/1 -> Matrix Concatenate/2
  Constant2/1 -> Matrix Concatenate2/2
  Gain/1 -> Matrix Concatenate2/1
  Matrix Concatenate3/1 -> Matrix Concatenate/3
  Gain1/1 -> Matrix Concatenate3/2
  Constant3/1 -> Matrix Concatenate3/3
  Constant1/1 -> Matrix Concatenate1/1
  Gain2/1 -> Matrix Concatenate1/3

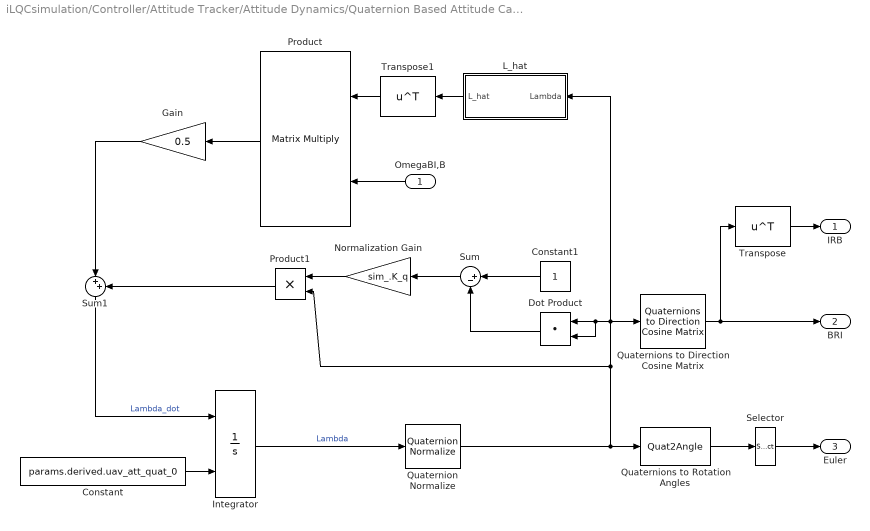
== system iLQCsimulation/Controller/Attitude Tracker/Attitude Dynamics/Quaternion Based Attitude Calculation ==
  OmegaBI,B : Inport
  Constant : Constant  Value=params.derived.uav_att_quat_0
  Constant1 : Constant
  Dot Product : DotProduct  InputSameDT=off  OutDataTypeStr=Inherit: Inherit via internal rule
  Gain : Gain  Gain=0.5
  Integrator : Integrator  InitialConditionSource=external
  L_hat : Subsystem
  Normalization Gain : Gain  Gain=sim_.K_q
  Product : Product  Multiplication=Matrix(*)  RndMeth=Zero
  Product1 : Product  RndMeth=Zero
  Quaternion Normalize : sharedutil/Quaternion Normalize  aMode=aMode
  Quaternions to Direction Cosine Matrix : sharedtransform/Quaternions to  Direction Cosine Matrix  aMode=aMode
  Quaternions to Rotation Angles : Quat2Angle
      settings: AttributesFormatString=Rotation Order: %<rotationOrder>
  Selector : Selector  InputPortWidth=3  IndexOptions=Index vector (dialog)  Indices=[3 2 1]  OutputSizes=1
  Sum : Sum  Inputs=|+-  InputSameDT=on  SaturateOnIntegerOverflow=on  OutDataTypeStr=Inherit: Same as first input
  Sum1 : Sum  Inputs=|++
  Transpose : Math  Operator=transpose  SignedPower=on
  Transpose1 : Math  Operator=transpose  SignedPower=on
  IRB : Outport  VectorParamsAs1DForOutWhenUnconnected=off
  BRI : Outport  Port=2  VectorParamsAs1DForOutWhenUnconnected=off
  Euler : Outport  Port=3  VectorParamsAs1DForOutWhenUnconnected=off
  wires:
  Constant/1 -> Integrator/2
  Quaternions to Rotation Angles/1 -> Selector/1
  Selector/1 -> Euler/1
  Integrator/1 -> Quaternion Normalize/1  "Lambda"
  Sum1/1 -> Integrator/1  "Lambda_dot"
  Quaternions to Direction Cosine Matrix/1 -> BRI/1, Transpose/1
  Transpose/1 -> IRB/1
  Dot Product/1 -> Sum/2
  Constant1/1 -> Sum/1
  L_hat/1(L_hat) -> Transpose1/1
  Transpose1/1 -> Product/1
  OmegaBI,B/1 -> Product/2
  Sum/1 -> Normalization Gain/1
  Product/1 -> Gain/1
  Gain/1 -> Sum1/1
  Normalization Gain/1 -> Product1/1
  Product1/1 -> Sum1/2
  Quaternion Normalize/1 -> Quaternions to Rotation Angles/1, Quaternions to Direction Cosine Matrix/1, Dot Product/1, Dot Product/2, L_hat/1(Lambda), Product1/2

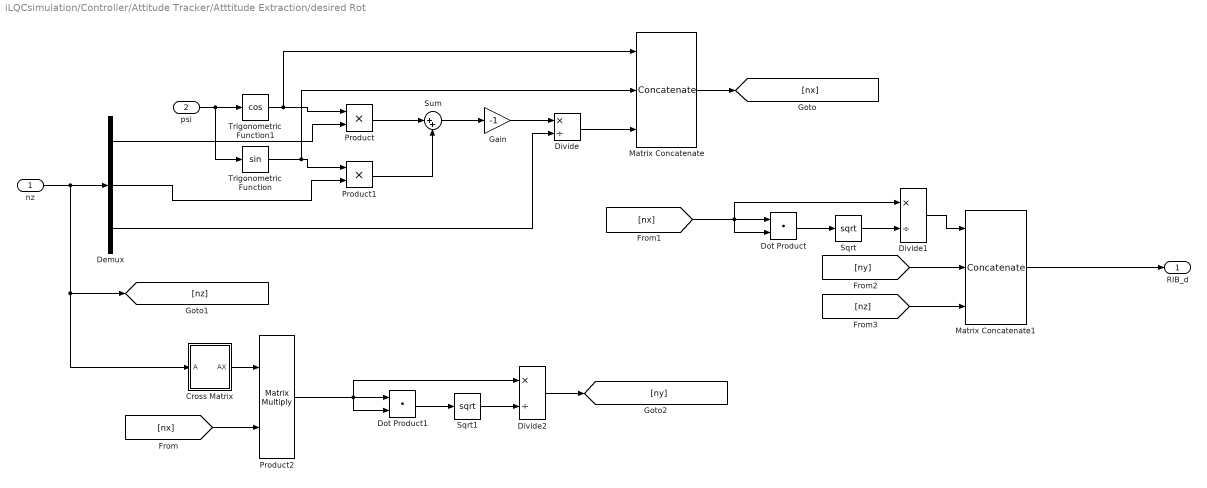
== system iLQCsimulation/Controller/Attitude Tracker/Atttitude Extraction/desired Rot ==
  nz : Inport
  psi : Inport  Port=2
  Cross Matrix : Subsystem
  Demux : Demux  Outputs=3
  Divide : Product  Inputs=*/
  Divide1 : Product  Inputs=*/
  Divide2 : Product  Inputs=*/
  Dot Product : DotProduct  OutDataTypeStr=Inherit: Inherit via internal rule
  Dot Product1 : DotProduct  OutDataTypeStr=Inherit: Inherit via internal rule
  Gain : Gain  Gain=-1
  Matrix Concatenate : Concatenate  NumInputs=3  Mode=Multidimensional array
  Matrix Concatenate1 : Concatenate  NumInputs=3  Mode=Multidimensional array  ConcatenateDimension=2
  Product : Product
  Product1 : Product
  Product2 : Product  Multiplication=Matrix(*)
  Sqrt : Sqrt
  Sqrt1 : Sqrt
  Sum : Sum  Inputs=|++
  Trigonometric Function : Trigonometry
  Trigonometric Function1 : Trigonometry  Operator=cos
  RIB_d : Outport  VectorParamsAs1DForOutWhenUnconnected=off
  wires:
  nz/1 -> Cross Matrix/1(A), [nz], Demux/1
  Demux/1 -> Product/2
  Demux/3 -> Divide/2
  psi/1 -> Trigonometric Function/1, Trigonometric Function1/1
  Trigonometric Function1/1 -> Matrix Concatenate/1, Product/1
  Trigonometric Function/1 -> Matrix Concatenate/2, Product1/1
  Demux/2 -> Product1/2
  Product/1 -> Sum/1
  Product1/1 -> Sum/2
  Sum/1 -> Gain/1
  Gain/1 -> Divide/1
  Divide/1 -> Matrix Concatenate/3
  Cross Matrix/1(AX) -> Product2/1
  [nx] -> Product2/2
  [ny] -> Matrix Concatenate1/2
  [nz] -> Matrix Concatenate1/3
  Product2/1 -> Divide2/1, Dot Product1/1, Dot Product1/2
  Dot Product1/1 -> Sqrt1/1
  Sqrt1/1 -> Divide2/2
  Divide2/1 -> [ny]
  Matrix Concatenate1/1 -> RIB_d/1
  Matrix Concatenate/1 -> [nx]
  Dot Product/1 -> Sqrt/1
  Divide1/1 -> Matrix Concatenate1/1
  [nx] -> Divide1/1, Dot Product/1, Dot Product/2
  Sqrt/1 -> Divide1/2

== system iLQCsimulation/Controller/Attitude Tracker/Atttitude Extraction/vee map ==
  skrew symmetric matrix : Inport
  Display2 : Display
  Display3 : Display
  Mux : Mux  Inputs=3
  Selector : Selector  NumberOfDimensions=2  InputPortWidth=3  IndexOptions=Index vector (dialog),Index vector (dialog)  Indices=3,2  OutputSizes=1,1
  Selector1 : Selector  NumberOfDimensions=2  InputPortWidth=3  IndexOptions=Index vector (dialog),Index vector (dialog)  Indices=1,3  OutputSizes=1,1
  Selector2 : Selector  NumberOfDimensions=2  InputPortWidth=3  IndexOptions=Index vector (dialog),Index vector (dialog)  Indices=2,1  OutputSizes=1,1
  phi : Outport  VectorParamsAs1DForOutWhenUnconnected=off
  wires:
  skrew symmetric matrix/1 -> Selector/1, Display3/1, Selector2/1, Selector1/1
  Mux/1 -> phi/1, Display2/1
  Selector/1 -> Mux/1
  Selector1/1 -> Mux/2
  Selector2/1 -> Mux/3

== system iLQCsimulation/Controller/Attitude Tracker/Attitude Dynamics/Quaternion Based Attitude Calculation/L_hat ==
  Lambda : Inport
  Create Diagonal Matrix1 : matrix_library/Create Diagonal Matrix
  Cross Matrix : Subsystem
  Gain : Gain  Gain=-1
  Gain1 : Gain  Gain=[1 1 1]
  Gain2 : Gain  Gain=-1
  Matrix Concatenate : Concatenate  Mode=Multidimensional array  ConcatenateDimension=2
  Selector : Selector  InputPortWidth=4  IndexOptions=Index vector (dialog)  Indices=[2 3 4]  OutputSizes=1
  Selector1 : Selector  InputPortWidth=4  IndexOptions=Index vector (dialog)  Indices=[1]  OutputSizes=1
  Sum : Sum  Inputs=|++
  L_hat : Outport  VectorParamsAs1DForOutWhenUnconnected=off
  wires:
  Lambda/1 -> Selector/1, Selector1/1
  Gain/1 -> Matrix Concatenate/1
  Matrix Concatenate/1 -> L_hat/1
  Cross Matrix/1(AX) -> Gain2/1  "LambdaX"
  Sum/1 -> Matrix Concatenate/2
  Selector1/1 -> Gain1/1
  Gain1/1 -> Create Diagonal Matrix1/1
  Selector/1 -> Cross Matrix/1(A), Gain/1
  Create Diagonal Matrix1/1 -> Sum/2
  Gain2/1 -> Sum/1

== system iLQCsimulation/Controller/Attitude Tracker/Atttitude Extraction/desired Rot/Cross Matrix ==
  A : Inport
  Constant1 : Constant  Value=0  VectorParams1D=off
  Constant2 : Constant  Value=0  VectorParams1D=off
  Constant3 : Constant  Value=0  VectorParams1D=off
  Demux2 : Demux  Outputs=3
  Gain : Gain  Gain=-1
  Gain1 : Gain  Gain=-1
  Gain2 : Gain  Gain=-1
  Matrix Concatenate : Concatenate  NumInputs=3  Mode=Multidimensional array  ConcatenateDimension=2
  Matrix Concatenate1 : Concatenate  NumInputs=3  Mode=Multidimensional array
  Matrix Concatenate2 : Concatenate  NumInputs=3  Mode=Multidimensional array
  Matrix Concatenate3 : Concatenate  NumInputs=3  Mode=Multidimensional array
  AX : Outport  VectorParamsAs1DForOutWhenUnconnected=off
  wires:
  A/1 -> Demux2/1
  Demux2/1 -> Gain1/1, Matrix Concatenate2/3  "r1"
  Demux2/2 -> Gain2/1, Matrix Concatenate3/1  "r2"
  Matrix Concatenate/1 -> AX/1
  Demux2/3 -> Gain/1, Matrix Concatenate1/2  "r3"
  Matrix Concatenate1/1 -> Matrix Concatenate/1
  Matrix Concatenate2/1 -> Matrix Concatenate/2
  Constant2/1 -> Matrix Concatenate2/2
  Gain/1 -> Matrix Concatenate2/1
  Matrix Concatenate3/1 -> Matrix Concatenate/3
  Gain1/1 -> Matrix Concatenate3/2
  Constant3/1 -> Matrix Concatenate3/3
  Constant1/1 -> Matrix Concatenate1/1
  Gain2/1 -> Matrix Concatenate1/3

== system iLQCsimulation/Controller/Attitude Tracker/Attitude Dynamics/Quaternion Based Attitude Calculation/L_hat/Cross Matrix ==
  A : Inport
  Constant1 : Constant  Value=0
  Constant2 : Constant  Value=0
  Constant3 : Constant  Value=0
  Demux2 : Demux  Outputs=3
  Gain : Gain  Gain=-1
  Gain1 : Gain  Gain=-1
  Gain2 : Gain  Gain=-1
  Matrix Concatenate : Concatenate  NumInputs=3  Mode=Multidimensional array  ConcatenateDimension=2
  Mux : Mux  Inputs=3
  Mux1 : Mux  Inputs=3
  Mux2 : Mux  Inputs=3
  AX : Outport  VectorParamsAs1DForOutWhenUnconnected=off
  wires:
  A/1 -> Demux2/1
  Demux2/1 -> Mux1/3, Gain1/1  "r1"
  Demux2/2 -> Mux2/1, Gain2/1  "r2"
  Matrix Concatenate/1 -> AX/1
  Demux2/3 -> Gain/1, Mux/2  "r3"
  Mux/1 -> Matrix Concatenate/1
  Mux1/1 -> Matrix Concatenate/2
  Constant2/1 -> Mux1/2
  Gain/1 -> Mux1/1
  Mux2/1 -> Matrix Concatenate/3
  Gain1/1 -> Mux2/2
  Constant3/1 -> Mux2/3
  Constant1/1 -> Mux/1
  Gain2/1 -> Mux/3

== stateflow chart iLQCsimulation/Controller/UDE controller /Chart ==
  state Initialization
    entry:
    index = initial_value;
    WayPoint_ni = reshape(WayPoint_n(:,index),3,1);
    WayPoint_Pi = reshape(WayPoint_P(:,index),3,1);
    WayPoint_vi =  WayPoint_v(index);
    flag=0;
    NUM_waypoints = max(size(WayPoint_v));
    position_error1 = 0;
  state Error
    during:
    if index<NUM_waypoints
    position_error1 = norm(Position-reshape(WayPoint_P(:,index+1),3,1));
    if position_error1<= WayPoint_v(index)*3
    flag=1;
    end
    else
    flag=0;
    end
  state INSIDE
    entry:
    index = index +1;
    WayPoint_ni = reshape(WayPoint_n(:,index),3,1);
    WayPoint_Pi = reshape(WayPoint_P(:,index),3,1);
    WayPoint_vi =  WayPoint_v(index);
    flag=0;
  (default) -> Initialization
  Initialization -> Error
  Error -> INSIDE : [flag==1]
  INSIDE -> Error : [flag==0]
  data: Position input; initial_value input; WayPoint_Pi output; WayPoint_ni output; WayPoint_P input; WayPoint_n input; index local; WayPoint_v input; WayPoint_vi output; flag local double size=1; position_error1 local; NUM_waypoints local
